simulink model "pai_lv6_simulink"  (Simulink 8.6)
settings: Solver=ode45  StartTime=0.0  StopTime=250.0  RelTol=1e-3
undefined symbols (not defined in the file): K1, K2
libraries: simulink x2
settings Model: Creator=korisnik15  LastModifiedBy=User
settings DataIOCC: SignalLoggingSaveFormat=Dataset
settings OptimizationCC: ExpressionDepthLimit=128
settings DebuggingCC: UnderspecifiedInitializationDetection=Simplified  MergeDetectMultiDrivingBlocksExec=error  SolverPrmCheckMsg=none  FcnCallInpInsideContextMsg=EnableAllAsError  StateNameClashWarn=none
settings GRTTargetCC: CombineOutputUpdateFcns=on  GRTInterface=off

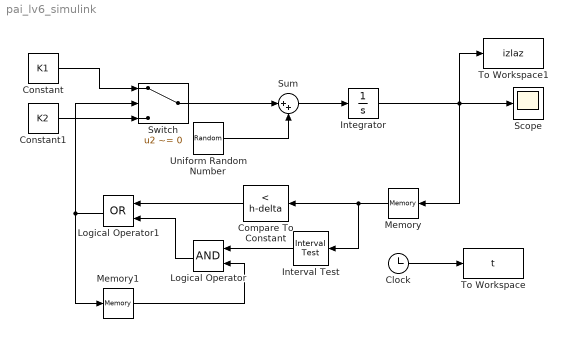
== system pai_lv6_simulink ==
  Clock : Clock
  Compare To Constant : simulink/Logic and Bit Operations/Compare To Constant  relop=<  const=h-delta  OutDataTypeStr=boolean
  Constant : Constant  Value=K1
  Constant1 : Constant  Value=K2
  Integrator : Integrator
  Interval Test : simulink/Logic and Bit Operations/Interval Test  IntervalClosedRight=on  uplimit=26  IntervalClosedLeft=on  lowlimit=-2  OutDataTypeStr=boolean
  Logical Operator : Logic  AllPortsSameDT=off  OutDataTypeStr=boolean
  Logical Operator1 : Logic  Operator=OR  AllPortsSameDT=off  OutDataTypeStr=boolean
  Memory : Memory
  Memory1 : Memory
  Scope : Scope
  Sum : Sum  Inputs=|++
  Switch : Switch  Criteria=u2 ~= 0
  To Workspace : ToWorkspace  VariableName=t  SampleTime=-1
  To Workspace1 : ToWorkspace  VariableName=izlaz  SampleTime=-1
  Uniform Random Number : UniformRandomNumber  Minimum=-0.3  Maximum=0.3  SampleTime=0.1
  wires:
  Switch/1 -> Sum/1
  Uniform Random Number/1 -> Sum/2
  Sum/1 -> Integrator/1
  Integrator/1 -> Memory/1, To Workspace1/1, Scope/1
  Interval Test/1 -> Logical Operator/1
  Memory/1 -> Compare To Constant/1, Interval Test/1
  Memory1/1 -> Logical Operator/2
  Logical Operator/1 -> Logical Operator1/2
  Compare To Constant/1 -> Logical Operator1/1
  Logical Operator1/1 -> Switch/2, Memory1/1
  Constant/1 -> Switch/1
  Constant1/1 -> Switch/3
  Clock/1 -> To Workspace/1
